simulink model "trajectory_data"  (R2023a)
settings: Solver=VariableStepAuto  StartTime=0.0  StopTime=2  RelTol=1e-3
libraries: robotcorelib x2, robotmaniplib x2
settings Model: Creator=ashu  LastModifiedBy=ashu
settings DataIOCC: ReturnWorkspaceOutputs=off

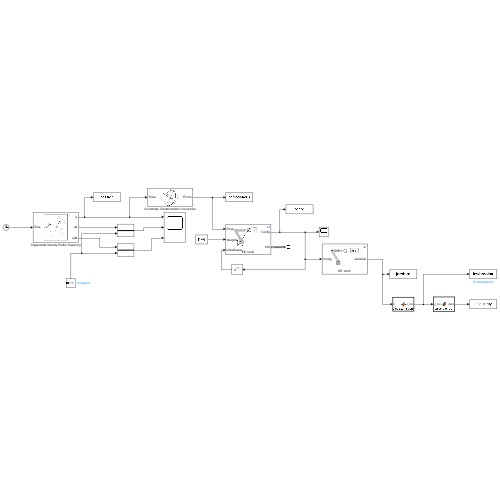
[thumbnail: Simulink's stored preview of the top-level diagram]
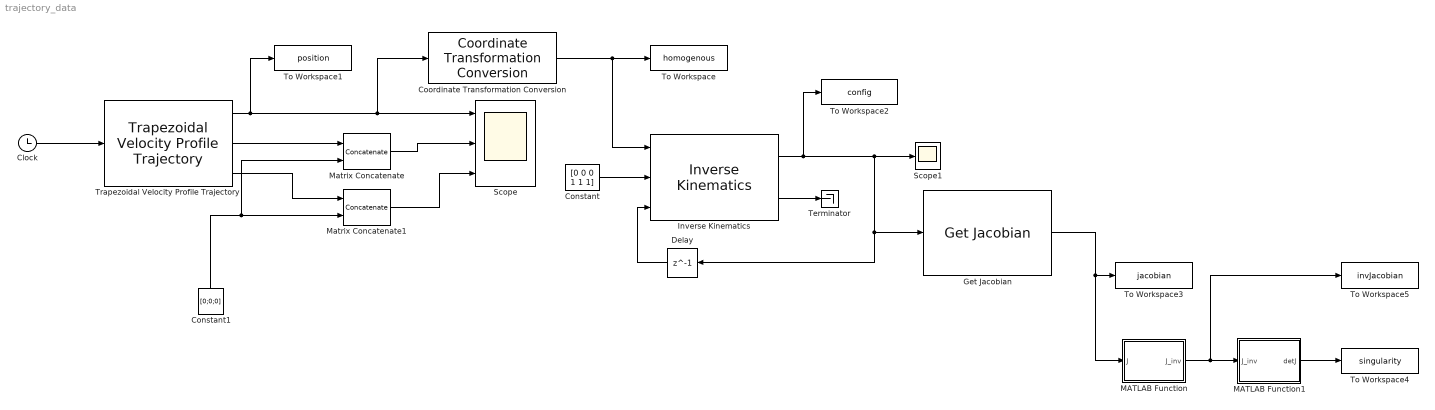
== system trajectory_data ==
  Clock : Clock
  Constant : Constant  Value=[0 0 0 1 1 1]
  Constant1 : Constant  Value=[0;0;0]
  Coordinate Transformation Conversion : robotcorelib/Coordinate Transformation Conversion  InputRepresentation=Translation Vector  InputEulerSequence=ZYX  ShowTrVecInputPort=on  OutputRepresentation=Homogeneous Transformation  OutputEulerSequence=ZYX  ShowTrVecOutputPort=on  SimulateUsing=Interpreted execution
  Delay : Delay  DelayLength=1
  Get Jacobian : robotmaniplib/Get Jacobian  RigidBodyTree=ur  EndEffector=tool0  SimulateUsing=Interpreted execution
  Inverse Kinematics : robotmaniplib/Inverse Kinematics  RigidBodyTree=ur  EndEffector=tool0  ShowInfo=on  SolverName=BFGS Gradient Projection  EnforceJointLimits=on  MaxIterations=1500  MaxTime=10  GradientTolerance=1e-7  SolutionTolerance=1e-6  StepTolerance=1e-14  ErrorChangeTolerance=1e-12  UseErrorDamping=on  DampingBias=0.0025  SimulateUsing=Interpreted execution
  MATLAB Function : MATLAB Function  TreatAsAtomicUnit=on
  MATLAB Function1 : MATLAB Function  TreatAsAtomicUnit=on
  Matrix Concatenate : Concatenate  ConcatenateDimension=2
  Matrix Concatenate1 : Concatenate  ConcatenateDimension=2
  Scope : Scope  NumInputPorts=3
  Scope1 : Scope
  Terminator : Terminator
  To Workspace : ToWorkspace  VariableName=homogenous  SampleTime=-1
      settings: Save2DSignal=2-D array (concatenate along first dimension)
  To Workspace1 : ToWorkspace  VariableName=position  SampleTime=-1
      settings: Save2DSignal=2-D array (concatenate along first dimension)
  To Workspace2 : ToWorkspace  VariableName=config  SampleTime=-1
      settings: Save2DSignal=2-D array (concatenate along first dimension)
  To Workspace3 : ToWorkspace  VariableName=jacobian  SampleTime=-1
      settings: Save2DSignal=2-D array (concatenate along first dimension)
  To Workspace4 : ToWorkspace  VariableName=singularity  SampleTime=-1
      settings: Save2DSignal=2-D array (concatenate along first dimension)
  To Workspace5 : ToWorkspace  VariableName=invJacobian  SampleTime=-1
      settings: Save2DSignal=2-D array (concatenate along first dimension)
  Trapezoidal Velocity Profile Trajectory : robotcorelib/Trapezoidal Velocity Profile Trajectory  WaypointSource=Internal  Waypoints=waypoints  NumParams=1  Parameter1=End Time  Parameter2=End Time  ParameterSource=Internal  PeakVelocity=[ 2; 2 ]  Acceleration=[ 1; 2 ]  EndTime=[ 1; 1 ]  AccelTime=[ 1; 2 ]  SimulateUsing=Interpreted execution
  wires:
  Clock/1 -> Trapezoidal Velocity Profile Trajectory/1
  Trapezoidal Velocity Profile Trajectory/1 -> Coordinate Transformation Conversion/1, Scope/1, To Workspace1/1
  Constant1/1 -> Matrix Concatenate1/2, Matrix Concatenate/2
  Trapezoidal Velocity Profile Trajectory/2 -> Matrix Concatenate/1
  Trapezoidal Velocity Profile Trajectory/3 -> Matrix Concatenate1/1
  Matrix Concatenate/1 -> Scope/2
  Matrix Concatenate1/1 -> Scope/3
  Coordinate Transformation Conversion/1 -> To Workspace/1, Inverse Kinematics/1
  Constant/1 -> Inverse Kinematics/2
  Inverse Kinematics/1 -> Delay/1, Get Jacobian/1, Scope1/1, To Workspace2/1
  Delay/1 -> Inverse Kinematics/3
  Inverse Kinematics/2 -> Terminator/1
  Get Jacobian/1 -> MATLAB Function/1(J), To Workspace3/1
  MATLAB Function/1(J_inv) -> To Workspace5/1, MATLAB Function1/1(J_inv)
  MATLAB Function1/1(detJ) -> To Workspace4/1

== matlab function trajectory_data/MATLAB Function ==
  data: J input; J_inv output
function J_inv  = calculate_inverse(J)
J_inv = inv(J);

== matlab function trajectory_data/MATLAB Function1 ==
  data: J_inv input; detJ output
function detJ = calculate_det(J_inv)
detJ = det(J_inv);
